simulink model "F450_SAS_joystick_FG_quaternion"  (R2022a)
settings: Solver=ode4  StartTime=0.0  StopTime=600  FixedStep=0.001  RelTol=1e-3
InitFcn:
  | F450_data
  | load Qtrim_hover.mat
values from neighbouring files (symbols this model uses):
  Alt_ground = 0    [F450_data.m]
undefined symbols (not defined in the file or in its folder): earthRadius, F, Light, MIL, Receive, Send, u0
libraries: simulink_extras x4, aerolibwind2 x3, aerolibfltsims x3, aerolibatmos2 x1, aerospace x1, vrlib x1, aerolibanimutils x1
settings Model: Creator=ADMIN  LastModifiedBy=USer
settings DebuggingCC: UnconnectedInputMsg=warning  UnconnectedOutputMsg=warning  UnconnectedLineMsg=warning
settings RTWCC: DLArmComputeVersion=19.05

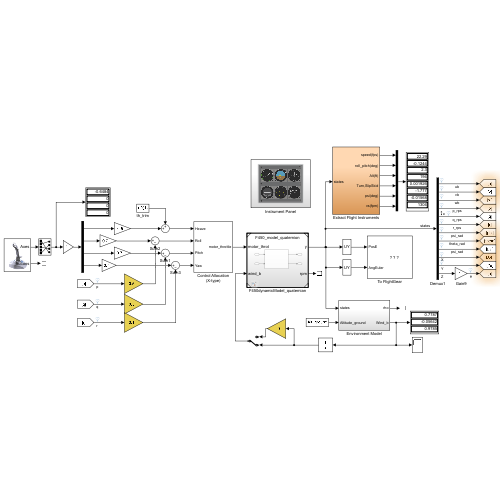
[thumbnail: Simulink's stored preview of the top-level diagram]
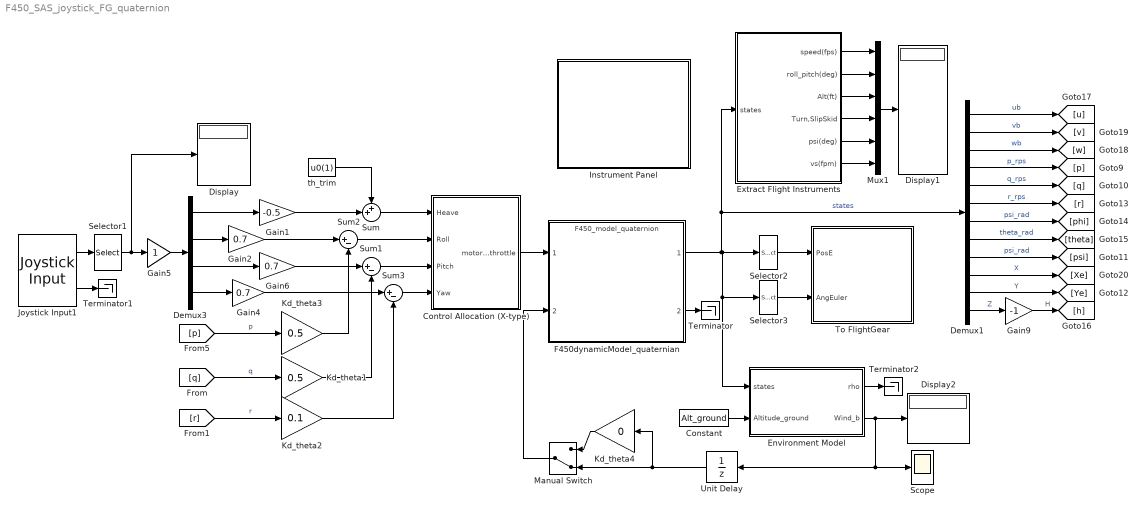
== system F450_SAS_joystick_FG_quaternion ==
  Constant : Constant  Value=Alt_ground
  Control Allocation (X-type) : Subsystem
  Demux1 : Demux  Outputs=12
  Demux3 : Demux
  Display : Display
  Display1 : Display
  Display2 : Display
  Environment Model : Subsystem
  Extract Flight Instruments : Subsystem
  F450dynamicModel_quaternian : ModelReference  ModelNameDialog=F450_model_quaternion.slx  SimulationMode=Normal  ModelReferenceVersion=10.81
  Gain1 : Gain  Gain=-0.5
  Gain2 : Gain  Gain=0.7
  Gain4 : Gain  Gain=0.7
  Gain5 : Gain
  Gain6 : Gain  Gain=0.7
  Gain9 : Gain  Gain=-1
  Instrument Panel : Subsystem
  Joystick Input1 : vrlib/Joystick Input  joyid=1  adjustports=on  forcefeed=off
  Kd_theta1 : Gain  Gain=0.5  SaturateOnIntegerOverflow=on  OutDataTypeStr=Inherit: Same as input  ParamDataTypeStr=Inherit: Same as input
  Kd_theta2 : Gain  Gain=0.1  SaturateOnIntegerOverflow=on  OutDataTypeStr=Inherit: Same as input  ParamDataTypeStr=Inherit: Same as input
  Kd_theta3 : Gain  Gain=0.5  SaturateOnIntegerOverflow=on  OutDataTypeStr=Inherit: Same as input  ParamDataTypeStr=Inherit: Same as input
  Kd_theta4 : Gain  Gain=0  SaturateOnIntegerOverflow=on  OutDataTypeStr=Inherit: Same as input  ParamDataTypeStr=Inherit: Same as input
  Manual Switch : ManualSwitch  CurrentSetting=0
  Mux1 : Mux  Inputs=6
  Scope : Scope
  Selector1 : Selector  InputPortWidth=5  IndexOptions=Index vector (dialog)  Indices=[2 5 3 1]  OutputSizes=1
  Selector2 : Selector  InputPortWidth=12  IndexOptions=Index vector (dialog)  Indices=10:12  OutputSizes=1
  Selector3 : Selector  InputPortWidth=12  IndexOptions=Index vector (dialog)  Indices=7:9  OutputSizes=1
  Sum : Sum  Inputs=++|
  Sum1 : Sum  Inputs=|+-  InputSameDT=on  SaturateOnIntegerOverflow=on  OutDataTypeStr=Inherit: Same as first input
  Sum2 : Sum  Inputs=|+-  InputSameDT=on  SaturateOnIntegerOverflow=on  OutDataTypeStr=Inherit: Same as first input
  Sum3 : Sum  Inputs=|+-  InputSameDT=on  SaturateOnIntegerOverflow=on  OutDataTypeStr=Inherit: Same as first input
  Terminator : Terminator
  Terminator1 : Terminator
  Terminator2 : Terminator
  To FlightGear : Subsystem
      mask Display: image('FlightGear.png'); % Use "Edit Image" on toolstrip to change.
  Unit Delay : UnitDelay  SampleTime=-1  HasFrameUpgradeWarning=on
  th_trim : Constant  Value=u0(1)  OutDataTypeStr=double
  wires:
  th_trim/1 -> Sum/1
  Demux3/3 -> Gain6/1
  Sum/1 -> Control Allocation (X-type)/1(Heave)
  Joystick Input1/2 -> Terminator1/1
  Joystick Input1/1 -> Selector1/1
  Selector1/1 -> Gain5/1, Display/1
  Demux3/1 -> Gain1/1
  Demux3/2 -> Gain2/1
  Demux3/4 -> Gain4/1
  F450dynamicModel_quaternian/1 -> Selector3/1, Environment Model/1(states), Selector2/1, Extract Flight Instruments/1(states), Demux1/1  "states"
  Demux1/7 -> [phi]  "psi_rad"
  Demux1/10 -> [Xe]  "X"
  Demux1/3 -> [w]  "wb"
  Demux1/8 -> [theta]  "theta_rad"
  Demux1/5 -> [q]  "q_rps"
  Demux1/1 -> [u]  "ub"
  Demux1/6 -> [r]  "r_rps"
  Gain9/1 -> [h]  "H"
  Demux1/12 -> Gain9/1  "Z"
  Demux1/11 -> [Ye]  "Y"
  Demux1/4 -> [p]  "p_rps"
  Demux1/9 -> [psi]  "psi_rad"
  Demux1/2 -> [v]  "vb"
  [q] -> Kd_theta1/1  "q"
  Sum1/1 -> Control Allocation (X-type)/3(Pitch)
  Sum2/1 -> Control Allocation (X-type)/2(Roll)
  [p] -> Kd_theta3/1  "p"
  Kd_theta1/1 -> Sum1/2
  Kd_theta3/1 -> Sum2/2
  Control Allocation (X-type)/1(motor_throttle) -> F450dynamicModel_quaternian/1
  Gain1/1 -> Sum/2
  Gain6/1 -> Sum1/1
  Gain2/1 -> Sum2/1
  F450dynamicModel_quaternian/2 -> Terminator/1
  Selector3/1 -> To FlightGear/2(AngEuler)
  Selector2/1 -> To FlightGear/1(PosE)
  Extract Flight Instruments/2(roll_pitch(deg)) -> Mux1/2
  Mux1/1 -> Display1/1
  Extract Flight Instruments/6(vs(fpm)) -> Mux1/6
  Extract Flight Instruments/3(Alt(ft)) -> Mux1/3
  Extract Flight Instruments/4(Turn,SlipSkid) -> Mux1/4
  Extract Flight Instruments/1(speed(fps)) -> Mux1/1
  Extract Flight Instruments/5(psi(deg)) -> Mux1/5
  Gain5/1 -> Demux3/1
  Constant/1 -> Environment Model/2(Altitude_ground)
  Environment Model/1(rho) -> Terminator2/1
  Environment Model/2(Wind_b) -> Scope/1, Unit Delay/1, Display2/1
  Unit Delay/1 -> Kd_theta4/1, Manual Switch/2
  Sum3/1 -> Control Allocation (X-type)/4(Yaw)
  Gain4/1 -> Sum3/1
  [r] -> Kd_theta2/1  "r"
  Kd_theta2/1 -> Sum3/2
  Manual Switch/1 -> F450dynamicModel_quaternian/2
  Kd_theta4/1 -> Manual Switch/1

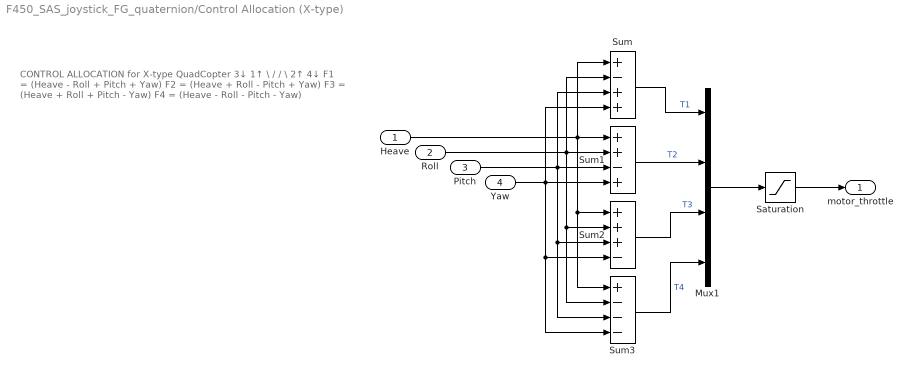
== system F450_SAS_joystick_FG_quaternion/Control Allocation (X-type) ==
  note: CONTROL ALLOCATION for X-type QuadCopter
      | 3↓ 1↑
      | \ /
      | / \
      | 2↑ 4↓
      | F1 = (Heave - Roll + Pitch + Yaw)
      | F2 = (Heave + Roll - Pitch + Yaw)
      | F3 = (Heave + Roll + Pitch - Yaw)
      | F4 = (Heave - Roll - Pitch - Yaw)
  Heave : Inport
  Roll : Inport  Port=2
  Pitch : Inport  Port=3
  Yaw : Inport  Port=4
  Mux1 : Mux
  Saturation : Saturate  UpperLimit=1  LowerLimit=0
      settings: AttributesFormatString=%<LowerLimit>~%<UpperLimit>
  Sum : Sum  Inputs=+-++
  Sum1 : Sum  Inputs=++-+
  Sum2 : Sum  Inputs=+++-
  Sum3 : Sum  Inputs=+---
  motor_throttle : Outport
  wires:
  Saturation/1 -> motor_throttle/1
  Yaw/1 -> Sum3/4, Sum2/4, Sum/4, Sum1/4
  Pitch/1 -> Sum3/3, Sum2/3, Sum/3, Sum1/3
  Sum3/1 -> Mux1/4  "T4"
  Mux1/1 -> Saturation/1
  Sum1/1 -> Mux1/2  "T2"
  Roll/1 -> Sum3/2, Sum2/2, Sum/2, Sum1/2
  Heave/1 -> Sum3/1, Sum2/1, Sum/1, Sum1/1
  Sum/1 -> Mux1/1  "T1"
  Sum2/1 -> Mux1/3  "T3"

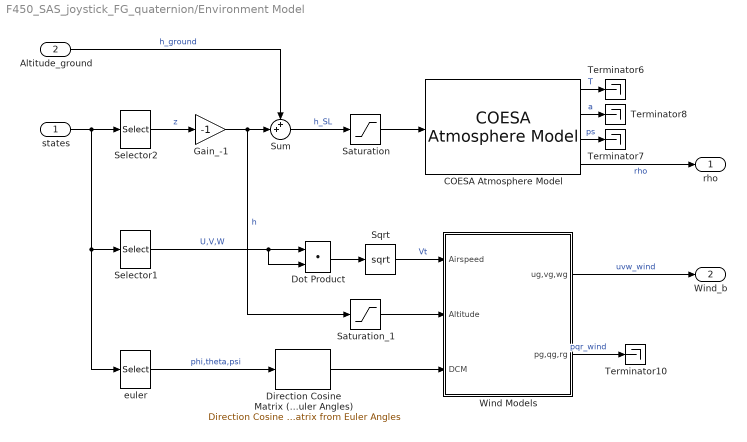
== system F450_SAS_joystick_FG_quaternion/Environment Model ==
  states : Inport
  Altitude_ground : Inport  Port=2
  COESA Atmosphere Model : aerolibatmos2/COESA Atmosphere Model  units=Metric (MKS)  spec=1976 COESA-extended U.S. Standard Atmosphere  model=Profile  profile_var=High temperature  profile_percent=1%  profile_alt=5 km (16404 ft)  envelope_var=High temperature  envelope_percent=1%  action=Warning
  Direction Cosine Matrix (Euler Angles) : aerospace/Axes Transformations/Direction Cosine Matrix from Euler Angles
      settings: SourceProductBaseCode=SL
  Dot Product : DotProduct  OutDataTypeStr=Inherit: Inherit via internal rule
  Gain_-1 : Gain  Gain=-1
  Saturation : Saturate  UpperLimit=100000  LowerLimit=0
  Saturation_1 : Saturate  UpperLimit=10000  LowerLimit=0
  Selector1 : Selector  InputPortWidth=12  IndexOptions=Index vector (dialog)  Indices=12  OutputSizes=1
  Selector2 : Selector  InputPortWidth=12  IndexOptions=Index vector (dialog)  Indices=12  OutputSizes=1
  Sqrt : Sqrt
  Sum : Sum  Inputs=++|
  Terminator{6..8,10} (4 alike) : Terminator
  Wind Models : Subsystem
  euler : Selector  InputPortWidth=12  IndexOptions=Index vector (dialog)  Indices=7:9  OutputSizes=1
  rho : Outport  VectorParamsAs1DForOutWhenUnconnected=off
  Wind_b : Outport  Port=2  VectorParamsAs1DForOutWhenUnconnected=off
  wires:
  Wind Models/1(ug,vg,wg) -> Wind_b/1  "uvw_wind"
  COESA Atmosphere Model/4 -> rho/1  "rho"
  Dot Product/1 -> Sqrt/1
  states/1 -> Selector2/1, euler/1, Selector1/1
  Sqrt/1 -> Wind Models/1(Airspeed)  "Vt"
  COESA Atmosphere Model/1 -> Terminator6/1  "T"
  Saturation_1/1 -> Wind Models/2(Altitude)
  COESA Atmosphere Model/2 -> Terminator8/1  "a"
  COESA Atmosphere Model/3 -> Terminator7/1  "ps"
  Wind Models/2(pg,qg,rg) -> Terminator10/1  "pqr_wind"
  Selector2/1 -> Gain_-1/1  "z"
  Sum/1 -> Saturation/1  "h_SL"
  Saturation/1 -> COESA Atmosphere Model/1
  Altitude_ground/1 -> Sum/1  "h_ground"
  Gain_-1/1 -> Saturation_1/1, Sum/2  "h"
  euler/1 -> Direction Cosine Matrix (Euler Angles)/1  "phi,theta,psi"
  Direction Cosine Matrix (Euler Angles)/1 -> Wind Models/3(DCM)
  Selector1/1 -> Dot Product/2, Dot Product/1  "U,V,W"

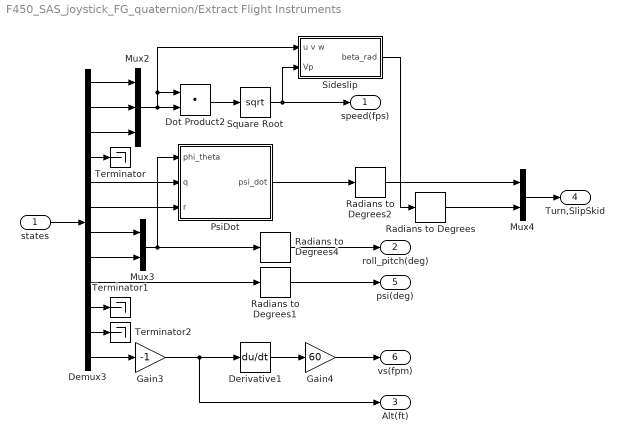
== system F450_SAS_joystick_FG_quaternion/Extract Flight Instruments ==
  states : Inport
  Demux3 : Demux  Outputs=12
  Derivative1 : Derivative
  Dot Product2 : DotProduct  OutDataTypeStr=Inherit: Inherit via internal rule
  Gain3 : Gain  Gain=-1
  Gain4 : Gain  Gain=60
  Mux2 : Mux  Inputs=3
  Mux3 : Mux  Inputs=2
  Mux4 : Mux  Inputs=2
  PsiDot : Subsystem
  Radians to Degrees{,1..2,4} (4 alike) : simulink_extras/Transformations/Radians to Degrees
  Sideslip : Subsystem
  Square Root : Sqrt
  Terminator : Terminator
  Terminator1 : Terminator
  Terminator2 : Terminator
  speed(fps) : Outport
  roll_pitch(deg) : Outport  Port=2
  Alt(ft) : Outport  Port=3
  Turn,SlipSkid : Outport  Port=4
  psi(deg) : Outport  Port=5
  vs(fpm) : Outport  Port=6
  wires:
  Radians to Degrees1/1 -> psi(deg)/1
  Derivative1/1 -> Gain4/1
  Mux2/1 -> Sideslip/1(u v w), Dot Product2/1, Dot Product2/2
  Radians to Degrees4/1 -> roll_pitch(deg)/1
  Mux3/1 -> Radians to Degrees4/1, PsiDot/1(phi_theta)
  Gain4/1 -> vs(fpm)/1
  Dot Product2/1 -> Square Root/1
  Gain3/1 -> Derivative1/1, Alt(ft)/1
  Demux3/12 -> Gain3/1
  Demux3/9 -> Radians to Degrees1/1
  Square Root/1 -> speed(fps)/1, Sideslip/2(Vp)
  states/1 -> Demux3/1
  Demux3/1 -> Mux2/1
  Demux3/2 -> Mux2/2
  Demux3/3 -> Mux2/3
  Demux3/7 -> Mux3/1
  Demux3/8 -> Mux3/2
  Demux3/5 -> PsiDot/2(q)
  Demux3/6 -> PsiDot/3(r)
  PsiDot/1(psi_dot) -> Radians to Degrees2/1
  Mux4/1 -> Turn,SlipSkid/1
  Demux3/4 -> Terminator/1
  Demux3/10 -> Terminator1/1
  Demux3/11 -> Terminator2/1
  Radians to Degrees2/1 -> Mux4/1
  Radians to Degrees/1 -> Mux4/2
  Sideslip/1(beta_rad) -> Radians to Degrees/1

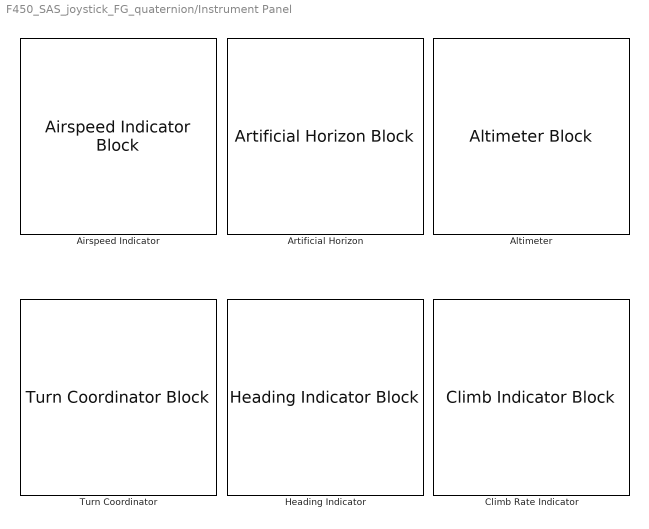
== system F450_SAS_joystick_FG_quaternion/Instrument Panel ==
  Airspeed Indicator : AirspeedIndicatorBlock  LabelPosition=Hide  ScaleMin=0  ScaleMax=450
  Altimeter : AltimeterBlock  LabelPosition=Hide
  Artificial Horizon : ArtificialHorizonBlock  LabelPosition=Hide
  Climb Rate Indicator : ClimbIndicatorBlock  LabelPosition=Hide  ScaleMax=16000
  Heading Indicator : HeadingIndicatorBlock  LabelPosition=Hide
  Turn Coordinator : TurnCoordinatorBlock  LabelPosition=Hide

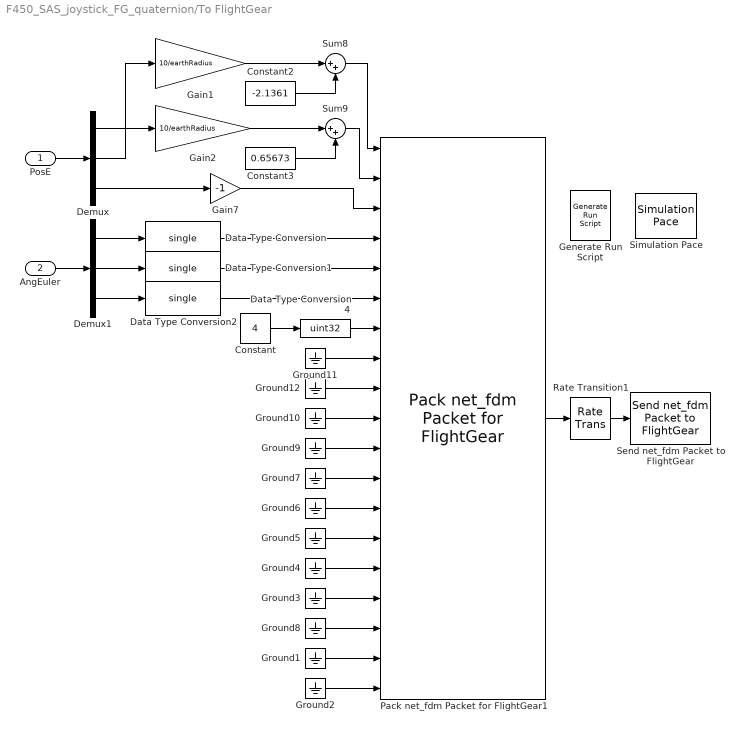
== system F450_SAS_joystick_FG_quaternion/To FlightGear ==
  PosE : Inport
  AngEuler : Inport  Port=2
  Constant : Constant  Value=4
  Constant2 : Constant  Value=-2.1361  VectorParams1D=off
  Constant3 : Constant  Value=0.65673  VectorParams1D=off
  Data Type Conversion : DataTypeConversion  OutDataTypeStr=single  RndMeth=Floor
  Data Type Conversion1 : DataTypeConversion  OutDataTypeStr=single  RndMeth=Floor
  Data Type Conversion2 : DataTypeConversion  OutDataTypeStr=single  RndMeth=Floor
  Data Type Conversion4 : DataTypeConversion  OutDataTypeStr=uint32  SaturateOnIntegerOverflow=off  RndMeth=Floor
  Demux : Demux  Outputs=3
  Demux1 : Demux  Outputs=3
  Gain1 : Gain  Gain=10/earthRadius
  Gain2 : Gain  Gain=10/earthRadius
  Gain7 : Gain  Gain=-1
  Generate Run Script : aerolibfltsims/Generate Run Script  Architecture=Default  dataFlow=Send-Receive  GeometryModelName=Rotor4  AirportId=KSF0  RunwayId=10L  InitialAltitude=0  InitialHeading=0  OffsetDistance=0  OffsetAzimuth=0  InstallScenery=off  DisableShaders=off  OriginAddress=127.0.0.1  DestinationPort=5502  OriginPort=5505  LocalAddress=127.0.0.1  OutputFileName=runfg.bat  FlightGearBaseDirectory=C:\Program Files\FlightGear 2016.1.2
  Ground{1..12} (12 alike) : Ground
  Pack net_fdm Packet for FlightGear1 : aerolibfltsims/Pack net_fdm Packet for FlightGear  FlightGearVersion=v2016.1  ShowPositionAttitudeInputs=on  ShowVelocityAccelerationInputs=off  ShowControlSurfacePositionInputs=off  ShowEngineFuelInputs=on  ShowLandingGearInputs=off  ShowEnvironmentInputs=off  SampleTime=0.001  packetVersion=24
      settings: SourceProductBaseCode=AE
  Rate Transition1 : RateTransition
  Send net_fdm Packet to FlightGear : aerolibfltsims/Send net_fdm Packet to FlightGear  DestinationIpAddress=127.0.0.1  DestinationPort=5502  LocalIpPort=-1  varLen=off  SampleTime=0.001
      settings: SourceProductBaseCode=AE
  Simulation Pace : aerolibanimutils/Simulation Pace  SimulationPace=1  SleepMode=MATLAB Thread  OutputPaceError=off  SampleTime=-1
      settings: AttributesFormatString=%<SimulationPace> sec/sec
  Sum8 : Sum  Inputs=|++
  Sum9 : Sum  Inputs=|++
  wires:
  Ground12/1 -> Pack net_fdm Packet for FlightGear1/9
  Ground3/1 -> Pack net_fdm Packet for FlightGear1/16
  Ground4/1 -> Pack net_fdm Packet for FlightGear1/15
  Ground5/1 -> Pack net_fdm Packet for FlightGear1/14
  Ground6/1 -> Pack net_fdm Packet for FlightGear1/13
  Ground7/1 -> Pack net_fdm Packet for FlightGear1/12
  Ground9/1 -> Pack net_fdm Packet for FlightGear1/11
  Ground10/1 -> Pack net_fdm Packet for FlightGear1/10
  Ground11/1 -> Pack net_fdm Packet for FlightGear1/8
  Ground2/1 -> Pack net_fdm Packet for FlightGear1/19
  Ground1/1 -> Pack net_fdm Packet for FlightGear1/18
  Ground8/1 -> Pack net_fdm Packet for FlightGear1/17
  Constant3/1 -> Sum9/2
  Constant2/1 -> Sum8/2
  Rate Transition1/1 -> Send net_fdm Packet to FlightGear/1
  Demux/2 -> Gain1/1
  Demux1/3 -> Data Type Conversion2/1
  Gain1/1 -> Sum8/1
  Gain2/1 -> Sum9/1
  Pack net_fdm Packet for FlightGear1/1 -> Rate Transition1/1
  Demux1/2 -> Data Type Conversion1/1
  Data Type Conversion4/1 -> Pack net_fdm Packet for FlightGear1/7
  Data Type Conversion2/1 -> Pack net_fdm Packet for FlightGear1/6
  Data Type Conversion1/1 -> Pack net_fdm Packet for FlightGear1/5
  Data Type Conversion/1 -> Pack net_fdm Packet for FlightGear1/4
  Sum8/1 -> Pack net_fdm Packet for FlightGear1/1
  Sum9/1 -> Pack net_fdm Packet for FlightGear1/2
  Demux/3 -> Gain7/1
  Constant/1 -> Data Type Conversion4/1
  Demux/1 -> Gain2/1
  Demux1/1 -> Data Type Conversion/1
  PosE/1 -> Demux/1
  AngEuler/1 -> Demux1/1
  Gain7/1 -> Pack net_fdm Packet for FlightGear1/3

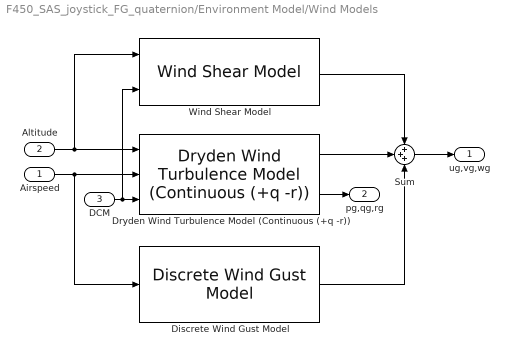
== system F450_SAS_joystick_FG_quaternion/Environment Model/Wind Models ==
  Airspeed : Inport  Unit=m/s
  Altitude : Inport  Port=2  Unit=meter
  DCM : Inport  Port=3
  Discrete Wind Gust Model : aerolibwind2/Discrete Wind Gust Model  units=Metric (MKS)  Gx=on  Gy=on  Gz=on  t_0=1  d_m=[120 120 80]  v_m=Wind_DiscreteGustAmp
  Dryden Wind Turbulence Model (Continuous (+q -r)) : aerolibwind2/Dryden Wind Turbulence Model  (Continuous (+q -r))  units=Metric (MKS)  spec=MIL-F-8785C  model=Continuous Dryden (+q -r)  W20=Wind_GustStrength  Wdeg=Wind_GustDirec  TurbProb=10^-2 - Light  L_high=533.4  Wingspan=1  ts=0.01  Seed=[23341 23342 23343 23344]  T_on=on
  Sum : Sum  Inputs=+++  InputSameDT=on  SaturateOnIntegerOverflow=on  OutDataTypeStr=Inherit: Same as first input
  Wind Shear Model : aerolibwind2/Wind Shear Model  units=Metric (MKS)  phase=Category C - Terminal Flight Phase  W_20=Wind_Strength  Wdeg=Wind_Direc
  ug,vg,wg : Outport  Unit=m/s  VectorParamsAs1DForOutWhenUnconnected=off
  pg,qg,rg : Outport  Port=2  Unit=rad/second  VectorParamsAs1DForOutWhenUnconnected=off
  wires:
  Sum/1 -> ug,vg,wg/1
  Airspeed/1 -> Dryden Wind Turbulence Model (Continuous (+q -r))/2, Discrete Wind Gust Model/1
  Dryden Wind Turbulence Model (Continuous (+q -r))/2 -> pg,qg,rg/1
  Discrete Wind Gust Model/1 -> Sum/3
  Dryden Wind Turbulence Model (Continuous (+q -r))/1 -> Sum/2
  DCM/1 -> Wind Shear Model/2, Dryden Wind Turbulence Model (Continuous (+q -r))/3
  Altitude/1 -> Wind Shear Model/1, Dryden Wind Turbulence Model (Continuous (+q -r))/1
  Wind Shear Model/1 -> Sum/1

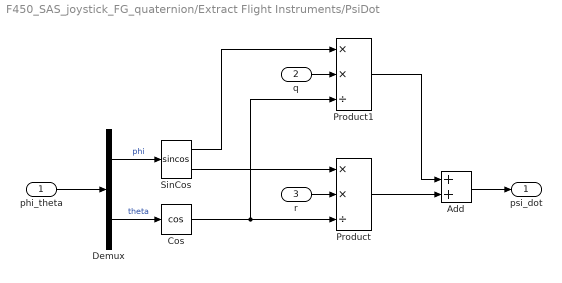
== system F450_SAS_joystick_FG_quaternion/Extract Flight Instruments/PsiDot ==
  phi_theta : Inport
  q : Inport  Port=2
  r : Inport  Port=3
  Add : Sum
  Cos : Trigonometry  Operator=cos
  Demux : Demux  Outputs=2
  Product : Product  Inputs=**/
  Product1 : Product  Inputs=**/
  SinCos : Trigonometry  Operator=sincos
  psi_dot : Outport
  wires:
  Demux/1 -> SinCos/1  "phi"
  Demux/2 -> Cos/1  "theta"
  Add/1 -> psi_dot/1
  Cos/1 -> Product/3, Product1/3
  q/1 -> Product1/2
  r/1 -> Product/2
  Product1/1 -> Add/1
  Product/1 -> Add/2
  SinCos/1 -> Product1/1
  SinCos/2 -> Product/1
  phi_theta/1 -> Demux/1

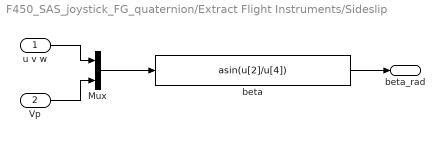
== system F450_SAS_joystick_FG_quaternion/Extract Flight Instruments/Sideslip ==
  u v w : Inport
  Vp : Inport  Port=2
  Mux : Mux  Inputs=2
  beta : Fcn  Expr=asin(u[2]/u[4])
  beta_rad : Outport  InitialOutput=0  VectorParamsAs1DForOutWhenUnconnected=off
  wires:
  Mux/1 -> beta/1
  beta/1 -> beta_rad/1
  Vp/1 -> Mux/2
  u v w/1 -> Mux/1
